simulink model "hw32f"  (R2017a)
settings: Solver=VariableStepAuto  StartTime=0.0  StopTime=10.0  RelTol=1e-3
undefined symbols (not defined in the file): sigbuilder_block
settings Model: Creator=Soutrik  LastModifiedBy=Soutrik

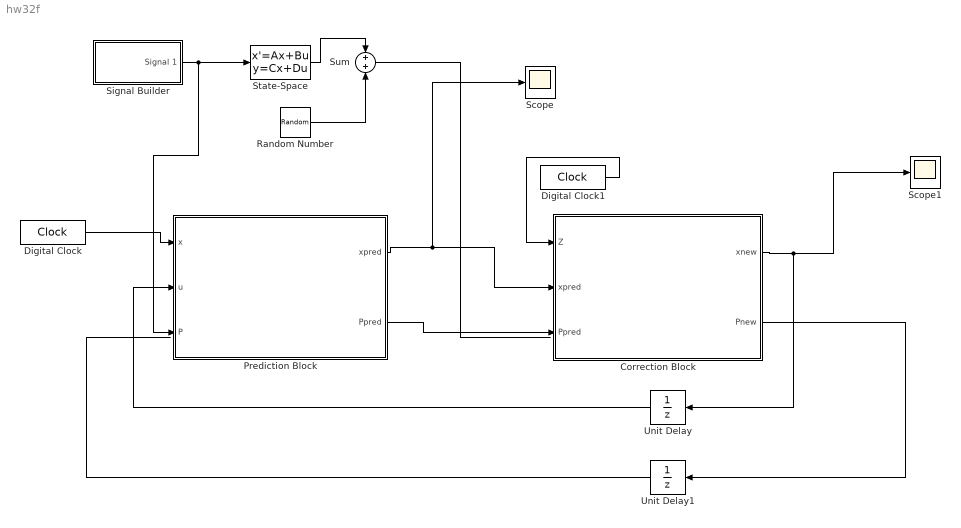
== system hw32f ==
  Correction Block : MATLAB Function  TreatAsAtomicUnit=on
  Digital Clock : DigitalClock  SampleTime=0.01
  Digital Clock1 : DigitalClock  SampleTime=0.01
  Prediction Block : MATLAB Function  TreatAsAtomicUnit=on
  Random Number : RandomNumber  Variance=[0.0001, 0.0000001, 0.00002, 0.00002]  SampleTime=0.01
  Scope : Scope
  Scope1 : Scope
  Signal Builder : Subsystem  Tag=STV Subsys  LoadFcn=sigbuilder_block('load');  StartFcn=sigbuilder_block('start');  StopFcn=sigbuilder_block('stop');  ClipboardFcn=sigbuilder_block('clipboard');  mask(Sigbuilder block){tuvar=[0:10]}
      mask help: Simulink:masks:SigbuilderBlock_MD
      mask init:
      | if ~strcmp(get_param(bdroot(gcbh),'SimulationStatus'),'stopped') tuvar = sigbuilder_block('maskInit'); end
      settings: CopyFcn=sigbuilder_block('copy');  DeleteFcn=sigbuilder_block('delete');  ModelCloseFcn=sigbuilder_block('modelClose');  PreSaveFcn=sigbuilder_block('preSave');  PauseFcn=sigbuilder_block('pause');  ContinueFcn=sigbuilder_block('continue');  NameChangeFcn=sigbuilder_block('namechange');  OpenFcn=sigbuilder_block('open',[300 184.875 550.5 400.125 ]);  CloseFcn=sigbuilder_block('close');
      mask Display: plot(0, 0, 100, 100,[2, 2, 32, 32, 2], [68, 8, 8, 68, 68],[32, 2], [38, 38], [32, 19, 2],[53, 60, 44], [32, 17, 17, 2],[16, 16, 31, 31]);txt = getActiveGroup(gcbh);text(2, 100, txt,'verticalAlignment', 'top');
  State-Space : StateSpace  A=|  B=|  C=|  D=[0;0;0;0];  X0=0
      A=|
      | [0 1.0000 0 0;
      | 0 -0.9965 0 -0.3000;
      | -0.3197 -0.5176 -0.0100 -0.7000;
      | 0 0 -0.0005 -0.9924];
      B=|
      | [ 0;
      | -0.0013;
      | 0.0001;
      | -0.0201];
      C=|
      | [0 0 0.9963 0.0862;
      | 0 0 -0.0001 0.0017;
      | 1.0000 0 0 0;
      | 0 1.0000 0 0];
  Sum : Sum  Inputs=2
  Unit Delay : UnitDelay  SampleTime=-1
  Unit Delay1 : UnitDelay  SampleTime=-1
  wires:
  Prediction Block/1(xpred) -> Scope/1, Correction Block/2(xpred)
  State-Space/1 -> Sum/1
  Random Number/1 -> Sum/2
  Signal Builder/1(Signal 1) -> Prediction Block/3(P), State-Space/1
  Sum/1 -> ?
  Correction Block/1(xnew) -> Scope1/1, Unit Delay/1
  Correction Block/2(Pnew) -> Unit Delay1/1
  Prediction Block/2(Ppred) -> Correction Block/3(Ppred)
  Unit Delay/1 -> Prediction Block/2(u)
  Unit Delay1/1 -> ?
  Digital Clock/1 -> Prediction Block/1(x)
  Digital Clock1/1 -> Correction Block/1(Z)

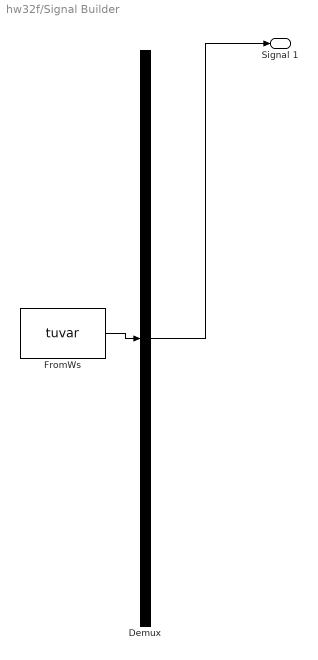
== system hw32f/Signal Builder ==
  Demux : Demux  Tag=STV Demux  Outputs=1
  FromWs : FromWorkspace  Tag=STV FromWs  VariableName=tuvar  SampleTime=0
      SigBuilderData=|
      | common.afterFinalStr = 'Extrapolate'
      | common.sampleTime = 0
      | dataSet.timeRange = [0 10]
      | dataSet.name = 'Group 1'
      | sbobj.Groups.Name = 'Group 1'
      | sbobj.Groups.Signals.Name = 'Signal 1'
      | sbobj.Groups.Signals.XData = [0 1.02 1.02 2.04 2.04 3.04 3.04 10]
      | sbobj.Groups.Signals.YData = [0 -0.002 50 50 -50 -50 0 0]
  Signal 1 : Outport  Tag=STV Outport
  wires:
  Demux/1 -> Signal 1/1
  FromWs/1 -> Demux/1

== matlab function hw32f/Correction Block ==
  data: Z input; xnew output; xpred input; Ppred input; Pnew output
function [xnew, Pnew] = corrector(Z,xpred,Ppred)
%xpred= A*x+B*U;
%Ppred=A*P*A'+Q;
R=diag([0.0001, 0.0000001, 0.00002, 0.00002]);
c = [0 0 0.9963 0.0862;
0 0 -0.0001 0.0017;
1.0000 0 0 0;
0 1.0000 0 0];
H=c;
K=Ppred*transpose(H)*inv(H*Ppred*(H)'+R);
Pnew=((eye(4)-K*H)*Ppred*transpose(eye(4)-K*H))+K*R*transpose(K);
xnew=xpred+K*(Z-H*xpred);

end

== matlab function hw32f/Prediction Block ==
  data: x input; u input; xpred output; P input; Ppred output
function [xpred, Ppred] = predict(x, u, P)
%xpred= A*x+B*U;
%Ppred=A*P*A'+Q;
b = [ 0;-0.0013;0.0001;-0.0201];
a =[0 1.0000 0 0;0 -0.9965 0 -0.3000;-0.3197 -0.5176 -0.0100 -0.7000;0 0 -0.0005 -0.9924];
Q = eye(4)*1;
P=1000*eye(4);
Ad=expm(a*0.01);
Bd=inv(a)*(Ad-eye(4))*b;
F=[-a Q;zeros(4,4) a'];
G=expm(F*0.01);
GLr=G(5:8,5:8);
Gur=G(1:4,5:8);
Qd=GLr'*Gur;
xpred=Ad*x+Bd*u;
Ppred=Ad*P*Ad'+Qd;
End
end
